simulink model "total"  (R2021a)
settings: Solver=VariableStepAuto  StartTime=0.0  StopTime=2.5  RelTol=1e-3
undefined symbols (not defined in the file or in its folder): Ion, Lithium
libraries: pid_lib x7, spsSeriesRLCBranchLib x4, spsMeanLib x4, spsACVoltageSourceLib x3, spsThreePhaseSeriesRLCBranchLib x3, spsGroundLib x2, spsabctodq0Lib x2, eePwmGenerator x2, spsOnDelayLib x2, spsBatteryLib x2, spsCurrentMeasurementLib x1, spsDiodeLib x1
settings Model: Creator=XieWHirlwind_TB  LastModifiedBy=XieWHirlwind_TB

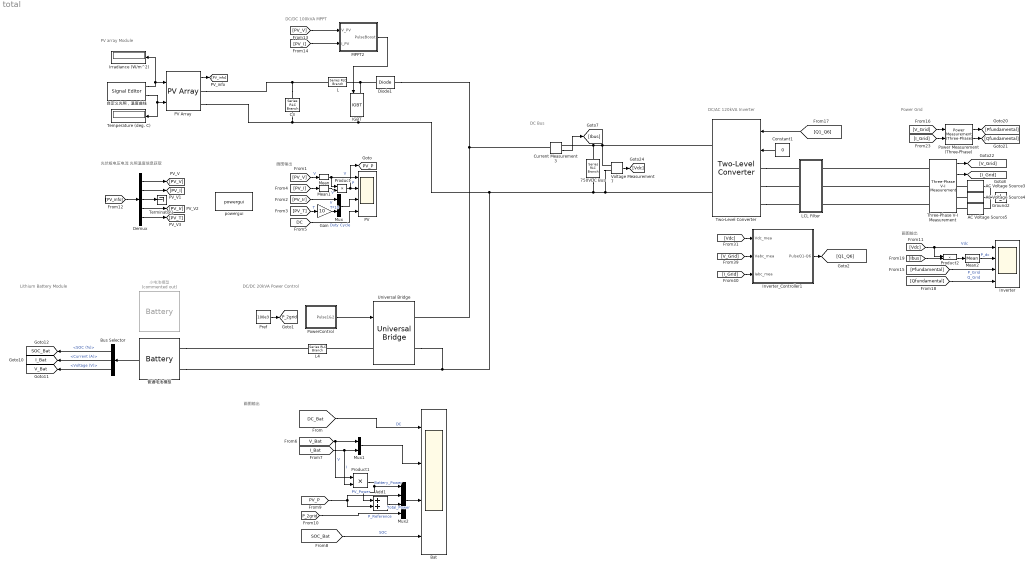
== system total ==
  note: 光伏板电压电流
      | 光照温度信息获取
  note: PV array Module
  note: 画图输出
  note: DC/DC 100kVA MPPT
  note: 画图输出
  note: DC/DC 20kVA Power Control
  note: Lithium Battery Module
  note: 画图输出
  note: DC/AC 120kVA Inverter
  note: Power Grid
  note: DC Bus
  750VDC Bus : spsSeriesRLCBranchLib/Series RLC Branch  LConnTagsString=__new0  RConnTagsString=__new0  BranchType=C  Resistance=1  Inductance=1e-3  SetiL0=off  InitialCurrent=0  Capacitance=470e-6  Setx0=on  InitialVoltage=0  Measurements=None
  AC Voltage Source3 : spsACVoltageSourceLib/AC Voltage Source  Amplitude=220*sqrt(2)  Phase=0  Frequency=50  SampleTime=0  Measurements=None  BusType=swing  Pref=10e3  Qref=0  Qmin=-inf  Qmax=+inf
  AC Voltage Source4 : spsACVoltageSourceLib/AC Voltage Source  Amplitude=220*sqrt(2)  Phase=-120  Frequency=50  SampleTime=0  Measurements=None  BusType=swing  Pref=10e3  Qref=0  Qmin=-inf  Qmax=+inf
  AC Voltage Source5 : spsACVoltageSourceLib/AC Voltage Source  Amplitude=220*sqrt(2)  Phase=120  Frequency=50  SampleTime=0  Measurements=None  BusType=swing  Pref=10e3  Qref=0  Qmin=-inf  Qmax=+inf
  Add1 : Sum
  Bat : Scope  NumInputPorts=4
  Bus Selector : BusSelector  OutputSignals=SOC (%),Current (A),Voltage (V)
  C3 : spsSeriesRLCBranchLib/Series RLC Branch  LConnTagsString=__new0  RConnTagsString=__new0  BranchType=C  Resistance=1.0  Inductance=1.0  SetiL0=off  InitialCurrent=0  Capacitance=470e-6  Setx0=off  InitialVoltage=0  Measurements=Branch voltage
  Constant1 : Constant  Value=0
  Current Measurement3 : spsCurrentMeasurementLib/Current Measurement  PhasorSimulation=off  OutputType=Complex  PSBequivalent=0
  Demux : Demux  Outputs=5
  Diode1 : spsDiodeLib/Diode  Ron=1e-3  Lon=0  Vf=0.7  IC=0  UseSnubber=off  Rs=inf  Cs=inf  Measurements=off
  Gain : Gain  Gain=10
  Ground2 : spsGroundLib/Ground  LConnTagsString=a
  IGBT : spsIGBTLib/IGBT  Ron=1e-3  Lon=0  Vf=0.7  Tf=1e-6  Tt=2e-6  IC=0  Rs=1e5  Cs=inf  Measurements=off
  Inverter : Scope  NumInputPorts=4
  Inverter_Controller1 : Subsystem  mask{Kp_Vdc_regulator=0.1, Ki_Vdc_regulator=10, Kp_Vdc_control=1, Ki_Vdc_control=1000, Kp_Q_regulator=1e-3, Ki_Q_regulator=1, Ts_Control=1e-4, L12=1e-3+3e-6, fsw=10e3, Vdc=750, Q_ref=5e3}
      mask prompts: Kp_Vdc_regulator "Kp"; Ki_Vdc_regulator "Ki"; Kp_Vdc_control "Kp"; Ki_Vdc_control "Ki"; Kp_Q_regulator "Kp"; Ki_Q_regulator "Ki"; Ts_Control "PI控制器控制周期(s)"; L12 "滤波器总串联电感(H)"; fsw "PWM频率(Hz)"; Vdc "直流母线电压(V)"; Q_ref "无功功率(VA)"
      mask DialogControl Container3 Prompt: 直流母线电压控制
      mask DialogControl Container4 Prompt: 电流环控制
      mask DialogControl Container5 Prompt: 无功功率控制
  Irradiance (W/m^2) : Display
      settings: Format=bank  Decimation=1000
  L : spsSeriesRLCBranchLib/Series RLC Branch  LConnTagsString=__new0  RConnTagsString=__new0  BranchType=RL  Resistance=0.0005  Inductance=1e-3  SetiL0=off  InitialCurrent=0  Capacitance=1e-6  Setx0=off  InitialVoltage=0  Measurements=None
  L4 : spsSeriesRLCBranchLib/Series RLC Branch  LConnTagsString=__new0  RConnTagsString=__new0  BranchType=RL  Resistance=0.001  Inductance=1e-3  SetiL0=off  InitialCurrent=0  Capacitance=1e-6  Setx0=off  InitialVoltage=0  Measurements=None
  LCL Filter : Subsystem  mask(LCL_Filter){Linv_LCL=1e-3, Lgrid_LCL=3e-6, Cap_LCL=1e-3, Rsnubber_LCL=0}
      mask prompts: Linv_LCL "逆变器侧电感"; Lgrid_LCL "电网侧电感"; Cap_LCL "并联电容"; Rsnubber_LCL "与电容串联的阻尼电阻"
  MPPT2 : Subsystem
  Mean : spsMeanLib/Mean  Freq=1e3  Vinit=0  Ts=1e-4
  Mean1 : spsMeanLib/Mean  Freq=1e3  Vinit=0  Ts=1e-4
  Mean2 : spsMeanLib/Mean  Freq=1/1e-3  Vinit=0  Ts=2e-6
  Mux : Mux  Inputs=2
  Mux1 : Mux  Inputs=2
  Mux2 : Mux
  PV : Scope  NumInputPorts=4
  PV Array : spsPVArrayLib/PV Array  Npar=45  Nser=10  PlotType=array @ 25 deg.C & specified irradiances  S_vec="[ 1000 800 350  100 ]"  Temp_C_vec="[ 45 25  ]"  ModuleName=A2Peak Power POWER ON P220-6x10  PlotWhenSelected=off  Pm=219.978  Ncell=60  Voc=36.72  Isc=7.98  Vm=30.3  Im=7.26  beta_Voc_pc=-0.35  alpha_Isc_pc=0.05  beta_Voc=-0.12852  alpha_Isc=0.00399  IL=8.0041  I0=1.8441e-10  nI=0.97472  Rsh=85.0716  Rs=0.25728  RobustModel=off  RobustCellTemperature=313.3991  BAL=on  Tc=1e-6  Tfilter=5e-5
  Power Measurement (Three-Phase) : eePowerMeasurement/Power Measurement (Three-Phase)  LabelModeActiveChoice=Discrete  F=50  K=[1]  Seq=Positive  Ts=1e-4
      settings: SourceProductBaseCode=PS
  PowerControl : Subsystem
  Pref : Constant  Value=100e3
  Product : Product
  Product1 : Product
  Product2 : Product
  Temperature (deg. C) : Display
      settings: Format=bank  Decimation=1000
  Terminator1 : Terminator
  Three-Phase V-I Measurement : spsThreePhaseVIMeasurementLib/Three-Phase V-I Measurement  VoltageMeasurement=phase-to-ground  SetLabelV=off  LabelV=Vabc  Vpu=off  VpuLL=off  CurrentMeasurement=yes  SetLabelI=off  LabelI=Iabc  Ipu=off  Pbase=100e6  Vbase=500e3  OutputType=Complex  PhasorSimulation=off  PSBequivalent=0
  Two-Level Converter : spsTwoLevelConverterLib/Two-Level Converter  ModelType=Switching devices  Ron=1e-3  Rs=1e6  Cs=inf  Vforward=[0,0]  Ron_Diode=1e-3  Rs_Diode=1e6  Cs_Diode=inf  Vf_Diode=1e-3  Rs_CurrentSource=inf
      settings: SourceProductBaseCode=PS
  Universal Bridge : spsUniversalBridgeLib/Universal Bridge  Arms=1  SnubberResistance=1e5  SnubberCapacitance=inf  Device=IGBT / Diodes  Ron=1e-3  Lon=0  ForwardVoltages="[0.7  0.7]"  ForwardVoltage=0  GTOparameters=[ 10e-6 , 20e-6 ]  IGBTparameters=[ 1e-6 , 2e-6 ]  Measurements=None  Measurements_2=None  converterType=Rectifier
  Voltage Measurement7 : spsVoltageMeasurementLib/Voltage Measurement  PhasorSimulation=off  OutputType=Complex  PSBequivalent=0
  powergui : spspowerguiLib/powergui  Priority=1  SimulationMode=Discrete  SampleTime=2e-6  frequency=60  Iterations=50  frequencyindice=0  Pbase=100e6  ErrMax=1e-4  UnitsV=kV  UnitsW=MW  buscounter=0  FunctionMessages=off  echomessages=off  EnableUseOfTLC=off  CurrentSourceSwitches=off  DisableSnubberDevices=off  DisableRonSwitches=off  DisableVfSwitches=off  DisplayEquations=off  AutomaticDiscreteSolvers=off  SolverType=Tustin/Backward Euler (TBE)  Interpol=off  ExternalGateDelay=off  methode=off  Ts=100  x0status=blocks  SPID=on  SwTol=0  HookPort=off  NonlinearTolerance=1e-4  nMaxIteration=100  ContinueOnMaxIteration=off  RestoreLinks=warning  ResistiveCurrentMeasurement=off  Frange=[0:2:500]  Ylog=off  Xlog=on  ShowGrid=off  save=off  variable=ZData  structure=0  ZoomFFT=off  StartTime=0.0  cycles=1  DisplayStyle=1  fundamental=60  FreqAxis=off  MaxFrequency=1000  frequencyindicesteady=1  RmsSteady=1  display=off
  小电池模型 : spsBatteryLib/Battery  Commented=on  BatType=Lithium-Ion  ShowTempParam=off  ThermalPreset=no  ShowAgeParam=off  NomV=640  NomQ=62.5/1000  SOC=50  Batt_Tr=30  PresetModel=off  MaxQ=62.5/100000  MinV=480  FullV=744.9518  Dis_rate=27.1739  R=0.1024  Normal_OP=56.5217/100000  expZone="[691.4469      3.070652/100000]"  current=[6.5 13 32.5]  Units=Time  Tci=20  NomT=20  T2=-30  MaxQ2=4.8  FullV2=7.1  Normal_OP2=5.655  expZone2="[6.58           1]"  Rca=0.6  ti=2000  Dp=0  Neq0=0  Tsim=1e6  Ta1=25  Qeol=5.4*0.9  Reol=0.013333*1.2  Char_age=[2.3478, 3]  Dis_age=[2.3478, 10]  N1=1500  N2=10500  N3=1000  N4=1400  Ta2=45  N5=950
  普通电池模型 : spsBatteryLib/Battery  BatType=Lithium-Ion  ShowTempParam=off  ThermalPreset=no  ShowAgeParam=off  NomV=640  NomQ=62.5  SOC=50  Batt_Tr=30  PresetModel=on  MaxQ=62.5  MinV=480  FullV=744.9518  Dis_rate=27.1739  R=0.1024  Normal_OP=56.5217  expZone="[691.4469      3.070652]"  current=[6.5 13 32.5]  Units=Time  Tci=20  NomT=20  T2=-30  MaxQ2=4.8  FullV2=7.1  Normal_OP2=5.655  expZone2="[6.58           1]"  Rca=0.6  ti=2000  Dp=0  Neq0=0  Tsim=1e6  Ta1=25  Qeol=5.4*0.9  Reol=0.013333*1.2  Char_age=[2.3478, 3]  Dis_age=[2.3478, 10]  N1=1500  N2=10500  N3=1000  N4=1400  Ta2=45  N5=950
  自定义光照，温度曲线 : SignalEditorBlockLib/Signal Editor  FileName=Irr_Temp_1.mat  ActiveScenario=Scenario  ActiveSignal=Temp  IsBus=off  OutputBusObjectStr=Bus: BusObject  SampleTime=0  ZeroCross=off  OutputAfterFinalValue=Setting to zero  Unit=inherit  PreserveSignalName=on
  tag scope: I_Bat=global, PV_P=global, P_2grid=global, SOC_Bat=global, V_Bat=global
  wires:
  Demux/4 -> [PV_Ir]
  [DC] -> PV/4  "Duty Cycle"
  [PV_V] -> MPPT2/1(V_PV)
  [PV_V] -> Mean/1  "V"
  Gain/1 -> Mux/2  "T*10"
  [PV_T] -> Gain/1  "T"
  Demux/5 -> [PV_T]
  Mean/1 -> Product/1, PV/1  "V"
  [PV_I] -> Mean1/1
  [PV_info] -> Demux/1
  MPPT2/1(PulseBoost) -> IGBT/1
  Demux/2 -> [PV_I]
  自定义光照，温度曲线/2 -> Temperature (deg. C)/1, PV Array/2
  Demux/3 -> Terminator1/1
  Mean1/1 -> Product/2  "V"
  Product/1 -> [PV_P], PV/2  "P"
  Demux/1 -> [PV_V]
  [PV_Ir] -> Mux/1  "Ir"
  自定义光照，温度曲线/1 -> Irradiance (W/m^2)/1, PV Array/1
  Mux/1 -> PV/3
  [PV_I] -> MPPT2/2(I_PV)
  PV Array/1 -> [PV_info]
  Pref/1 -> [P_2grid]
  PowerControl/1(Pulse1&2) -> Universal Bridge/1
  Mux1/1 -> Bat/2
  [PV_P] -> Add1/2, Mux2/2  "PV_Power"
  [I_Bat] -> Product1/2, Mux1/2  "I"
  [V_Bat] -> Mux1/1, Product1/1  "V"
  [DC_Bat] -> Bat/1  "DC"
  Bus Selector/3 -> [V_Bat]  "<Voltage (V)>"
  Bus Selector/1 -> [SOC_Bat]  "<SOC (%)>"
  普通电池模型/1 -> Bus Selector/1
  Product1/1 -> Add1/1, Mux2/1  "Battery_Power"
  Bus Selector/2 -> [I_Bat]  "<Current (A)>"
  [SOC_Bat] -> Bat/4  "SOC"
  [P_2grid] -> Mux2/4  "P_Reference"
  Mux2/1 -> Bat/3
  Add1/1 -> Mux2/3  "Total_Power"
  Mean2/1 -> Inverter/2  "P_dc"
  Product2/1 -> Mean2/1
  Three-Phase V-I Measurement/1 -> [V_Grid]
  [Vdc] -> Inverter_Controller1/1(Vdc_mea)
  Power Measurement (Three-Phase)/1 -> [Pfundamental]
  [Vdc] -> Inverter/1, Product2/1  "Vdc"
  [I_Grid] -> Power Measurement (Three-Phase)/2
  Three-Phase V-I Measurement/2 -> [I_Grid]
  [Qfundamental] -> Inverter/4  "Q_Grid"
  Power Measurement (Three-Phase)/2 -> [Qfundamental]
  [I_Grid] -> Inverter_Controller1/3(Iabc_mea)
  [Pfundamental] -> Inverter/3  "P_Grid"
  [Q1_Q6] -> Two-Level Converter/1
  [V_Grid] -> Power Measurement (Three-Phase)/1
  Constant1/1 -> Two-Level Converter/2
  [V_Grid] -> Inverter_Controller1/2(Vabc_mea)
  Inverter_Controller1/1(PulseQ1-Q6) -> [Q1_Q6]
  [Ibus] -> Product2/2
  Voltage Measurement7/1 -> [Vdc]
  Current Measurement3/1 -> [Ibus]
  connections:
  Diode1/LConn1 -- L/RConn1 -- IGBT/LConn1
  C3/LConn1 -- PV Array/RConn1 -- L/LConn1
  Universal Bridge/LConn1 -- L4/RConn1
  普通电池模型/LConn1 -- L4/LConn1
  Ground2/LConn1 -- AC Voltage Source5/LConn1 -- AC Voltage Source4/LConn1 -- AC Voltage Source3/LConn1
  Two-Level Converter/LConn3 -- LCL Filter/LConn3
  AC Voltage Source5/RConn1 -- Three-Phase V-I Measurement/RConn3
  Two-Level Converter/LConn2 -- LCL Filter/LConn2
  AC Voltage Source3/RConn1 -- Three-Phase V-I Measurement/RConn1
  Three-Phase V-I Measurement/LConn1 -- LCL Filter/RConn1
  Three-Phase V-I Measurement/LConn2 -- LCL Filter/RConn2
  Three-Phase V-I Measurement/LConn3 -- LCL Filter/RConn3
  AC Voltage Source4/RConn1 -- Three-Phase V-I Measurement/RConn2
  Two-Level Converter/LConn1 -- LCL Filter/LConn1
  PV Array/RConn2 -- Two-Level Converter/RConn2 -- Voltage Measurement7/LConn2 -- 750VDC Bus/RConn1 -- 普通电池模型/LConn2 -- Universal Bridge/RConn2 -- IGBT/RConn1 -- C3/RConn1
  Voltage Measurement7/LConn1 -- 750VDC Bus/LConn1 -- Current Measurement3/RConn1 -- Two-Level Converter/RConn1
  Current Measurement3/LConn1 -- Diode1/RConn1 -- Universal Bridge/RConn1

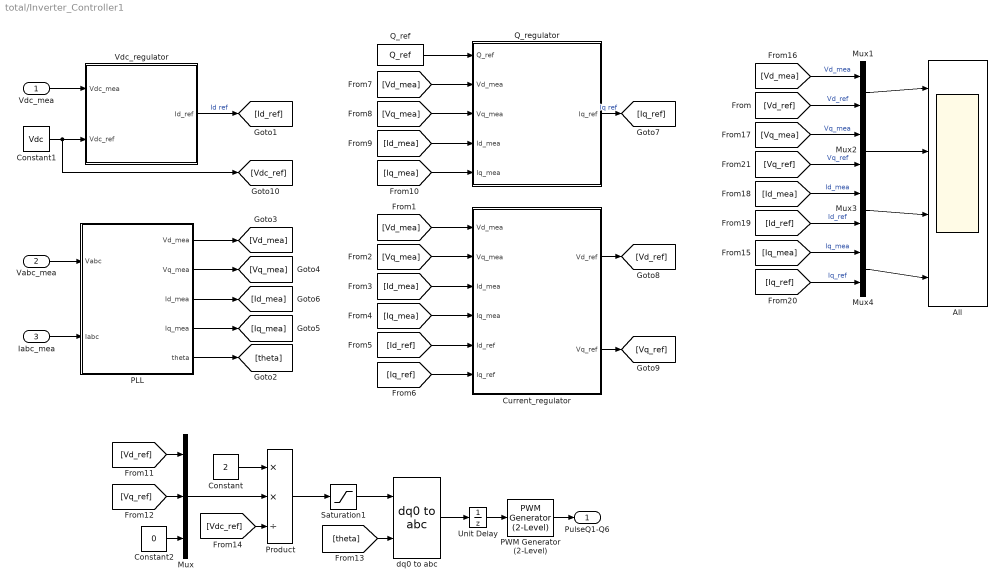
== system total/Inverter_Controller1 ==
  Vdc_mea : Inport
  Vabc_mea : Inport  Port=2
  Iabc_mea : Inport  Port=3
  All : Scope  NumInputPorts=4
  Constant : Constant  Value=2
  Constant1 : Constant  Value=Vdc
  Constant2 : Constant  Value=0
  Current_regulator : Subsystem
  Mux : Mux  Inputs=3
  Mux{1..4} (4 alike) : Mux  Inputs=2
  PLL : Subsystem
  PWM Generator (2-Level) : spsPWMGenerator2LevelLib/PWM Generator (2-Level)  ModulatorType=Three-phase bridge (6 pulses)  ModulatorMode=Unsynchronized  Fc=fsw  Pc=90  nF=27  MinMax="[ -1  1 ]"  SamplingTechnique=Asymmetrical regular (double edge)  ModulatingSignals=off  m=0.8  Freq=60  Phase=0  Ts=1e-6  ShowCarrierOutport=off
  Product : Product  Inputs=**/
  Q_ref : Constant  Value=Q_ref
  Q_regulator : Subsystem
  Saturation1 : Saturate  UpperLimit=2  LowerLimit=-2
  Unit Delay : UnitDelay  SampleTime=Ts_Control  HasFrameUpgradeWarning=on
  Vdc_regulator : Subsystem
  dq0 to abc : spsdq0toabcLib/dq0 to abc  Alignment=90 degrees behind phase A axis
  PulseQ1-Q6 : Outport
  wires:
  Constant1/1 -> [Vdc_ref], Vdc_regulator/2(Vdc_ref)
  Vabc_mea/1 -> PLL/1(Vabc)
  Iabc_mea/1 -> PLL/2(Iabc)
  PWM Generator (2-Level)/1 -> PulseQ1-Q6/1
  Saturation1/1 -> dq0 to abc/1
  dq0 to abc/1 -> Unit Delay/1
  Product/1 -> Saturation1/1
  Unit Delay/1 -> PWM Generator (2-Level)/1
  Vdc_mea/1 -> Vdc_regulator/1(Vdc_mea)
  Q_ref/1 -> Q_regulator/1(Q_ref)
  Constant/1 -> Product/1
  [Vdc_ref] -> Product/3
  Vdc_regulator/1(Id_ref) -> [Id_ref]  "Id ref"
  PLL/5(theta) -> [theta]
  PLL/1(Vd_mea) -> [Vd_mea]
  PLL/2(Vq_mea) -> [Vq_mea]
  PLL/3(Id_mea) -> [Id_mea]
  PLL/4(Iq_mea) -> [Iq_mea]
  [Vd_mea] -> Current_regulator/1(Vd_mea)
  [Vq_mea] -> Current_regulator/2(Vq_mea)
  [Id_mea] -> Current_regulator/3(Id_mea)
  [Iq_mea] -> Current_regulator/4(Iq_mea)
  [Id_ref] -> Current_regulator/5(Id_ref)
  Q_regulator/1(Iq_ref) -> [Iq_ref]  "Iq ref"
  [Iq_ref] -> Current_regulator/6(Iq_ref)
  [Vd_mea] -> Q_regulator/2(Vd_mea)
  [Vq_mea] -> Q_regulator/3(Vq_mea)
  [Id_mea] -> Q_regulator/4(Id_mea)
  [Iq_mea] -> Q_regulator/5(Iq_mea)
  Current_regulator/1(Vd_ref) -> [Vd_ref]
  Current_regulator/2(Vq_ref) -> [Vq_ref]
  [Vd_ref] -> Mux/1
  [Vq_ref] -> Mux/2
  Constant2/1 -> Mux/3
  Mux/1 -> Product/2
  [theta] -> dq0 to abc/2
  [Vd_mea] -> Mux1/1  "Vd_mea"
  [Vd_ref] -> Mux1/2  "Vd_ref"
  [Vq_mea] -> Mux2/1  "Vq_mea"
  [Vq_ref] -> Mux2/2  "Vq_ref"
  [Id_mea] -> Mux3/1  "Id_mea"
  [Id_ref] -> Mux3/2  "Id_ref"
  [Iq_mea] -> Mux4/1  "Iq_mea"
  [Iq_ref] -> Mux4/2  "Iq_ref"
  Mux2/1 -> All/2
  Mux1/1 -> All/1
  Mux3/1 -> All/3
  Mux4/1 -> All/4

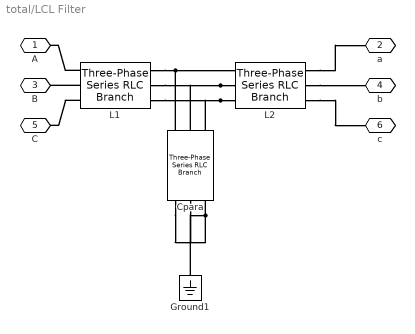
== system total/LCL Filter ==
  Cpara : spsThreePhaseSeriesRLCBranchLib/Three-Phase Series RLC Branch  LConnTagsString=A|B|C  RConnTagsString=A|B|C  BranchType=RC  Resistance=Rsnubber_LCL  Inductance=1e-3  Capacitance=Cap_LCL  Measurements=None
  Ground1 : spsGroundLib/Ground  LConnTagsString=a
  L1 : spsThreePhaseSeriesRLCBranchLib/Three-Phase Series RLC Branch  LConnTagsString=A|B|C  RConnTagsString=A|B|C  BranchType=L  Resistance=1  Inductance=Linv_LCL  Capacitance=1e-6  Measurements=None
  L2 : spsThreePhaseSeriesRLCBranchLib/Three-Phase Series RLC Branch  LConnTagsString=A|B|C  RConnTagsString=A|B|C  BranchType=L  Resistance=1  Inductance=Lgrid_LCL  Capacitance=1e-6  Measurements=None
  A : PMIOPort  Side=Left
  a : PMIOPort  Port=2  Side=Right
  B : PMIOPort  Port=3  Side=Left
  b : PMIOPort  Port=4  Side=Right
  C : PMIOPort  Port=5  Side=Left
  c : PMIOPort  Port=6  Side=Right
  connections:
  L2/RConn2 -- b/RConn1
  L2/LConn2 -- L1/RConn2 -- Cpara/LConn2
  L2/LConn3 -- L1/RConn3 -- Cpara/LConn3
  Cpara/RConn3 -- Cpara/RConn2 -- Ground1/LConn1 -- Cpara/RConn1
  L1/LConn3 -- C/RConn1
  L1/LConn1 -- A/RConn1
  L2/RConn1 -- a/RConn1
  L1/LConn2 -- B/RConn1
  L2/RConn3 -- c/RConn1
  L1/RConn1 -- L2/LConn1 -- Cpara/LConn1

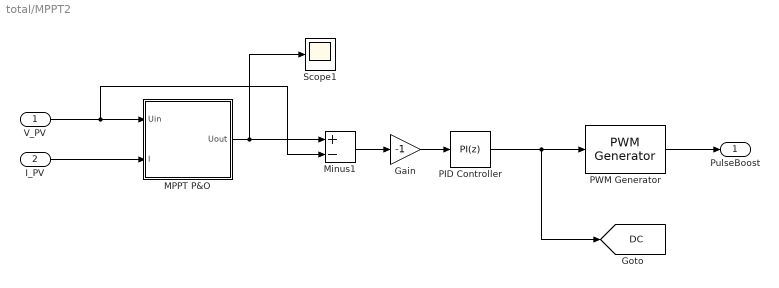
== system total/MPPT2 ==
  V_PV : Inport
  I_PV : Inport  Port=2
  Gain : Gain  Gain=-1
  MPPT P&O : Subsystem
  Minus1 : Sum  Inputs=+-
  PID Controller : pid_lib/PID Controller  Controller=PI  Form=Parallel  TimeDomain=Discrete-time  UseExternalTs=off  SampleTime=1e-4  IntegratorMethod=Forward Euler  FilterMethod=Forward Euler  ControllerParametersSource=internal  P=0.001  I=0.1  D=0  UseFilter=on  N=100  TunerSelectOption=Transfer Function Based (PID Tuner App)  InitialConditionSource=internal  InitialConditionForIntegrator=0  InitialConditionForFilter=0  DifferentiatorICPrevScaledInput=0  ExternalReset=none  TrackingMode=off  Kt=1  LimitOutput=on  SatLimitsSource=internal  UpperSaturationLimit=1  LowerSaturationLimit=0  LinearizeAsGain=on  AntiWindupMode=none  Kb=1  POutMin=[]  POutMax=[]  IOutMin=[]  IOutMax=[]  DOutMin=[]  DOutMax=[]  NOutMin=[]  NOutMax=[]  SumOutMin=[]  SumOutMax=[]  SaturationOutMin=[]  SaturationOutMax=[]  PParamMin=[]  PParamMax=[]  IParamMin=[]  IParamMax=[]  DParamMin=[]  DParamMax=[]  NParamMin=[]  NParamMax=[]  KbParamMin=[]  KbParamMax=[]  KtParamMin=[]  KtParamMax=[]  KbOutMin=[]  KbOutMax=[]  KtOutMin=[]  KtOutMax=[]  IntegratorOutMin=[]  IntegratorOutMax=[]  FilterOutMin=[]  FilterOutMax=[]  SumI1OutMin=[]  SumI1OutMax=[]  SumI2OutMin=[]  SumI2OutMax=[]  SumI3OutMin=[]  SumI3OutMax=[]  SumI4OutMin=[]  SumI4OutMax=[]  SumDOutMin=[]  SumDOutMax=[]  DifferentiatorOutMin=[]  DifferentiatorOutMax=[]  FilterDiffOutCoefMin=[]  FilterDiffOutCoefMax=[]  ReciprocalOutMin=[]  ReciprocalOutMax=[]  SumDenOutMin=[]  SumDenOutMax=[]  SumNumOutMin=[]  SumNumOutMax=[]  DivideOutMin=[]  DivideOutMax=[]  UdiffTsProdOutMin=[]  UdiffTsProdOutMax=[]  NTsProdOutMin=[]  NTsProdOutMax=[]  UintegralTsProdOutMin=[]  UintegralTsProdOutMax=[]  UngainTsProdOutMin=[]  UngainTsProdOutMax=[]  IntegratorContinuousStateAttributes=''  IntegratorStateMustResolveToSignalObject=off  IntegratorRTWStateStorageClass=Auto  FilterContinuousStateAttributes=''  FilterStateMustResolveToSignalObject=off  FilterRTWStateStorageClass=Auto  ParallelPVariant=InternalParameters  IdealPVariant=Disabled  IVariant=InternalParameters  DVariant=Disabled  IntegratorVariant=Discrete  SatVariant=Enabled  AWVariant=Passthrough  PCopyVariant=Disabled  TRVariant=Disabled  FdbkBlocksVariant=Forward  IdealPFdbkVariant=Disabled  SatFdbkVariant=Disabled  DerivativeFilterVariant=Disabled  NVariant=Disabled  NCopyVariant=Disabled_SignalSpec  FilterICVariant=Disabled  IntegratorICVariant=InternalICs  ExternalResetVariant=Disabled  TRSumVariant=Passthrough  SumFdbkVariant=Disabled  SumVariant=Sum_PI  TsampFilterVariant=InternalTs  TsampNgainVariant=Passthrough  TsampIntegralVariant=Passthrough  ExternalSaturationOutDataTypeStr=Inherit: Same as second input
  PWM Generator : eePwmGenerator/PWM Generator  CarrCount=Up  Tper=1e-4  Ts=2e-6
  Scope1 : Scope
  PulseBoost : Outport
  tag scope: DC=global
  wires:
  PWM Generator/1 -> PulseBoost/1
  I_PV/1 -> MPPT P&O/2(I)
  V_PV/1 -> Minus1/2, MPPT P&O/1(Uin)
  MPPT P&O/1(Uout) -> Minus1/1, Scope1/1
  Minus1/1 -> Gain/1
  PID Controller/1 -> [DC], PWM Generator/1
  Gain/1 -> PID Controller/1

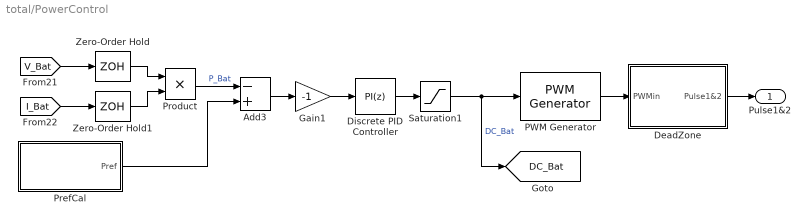
== system total/PowerControl ==
  Add3 : Sum  Inputs=-+
  DeadZone : Subsystem
  Discrete PID Controller : pid_lib/PID Controller  Controller=PI  Form=Parallel  TimeDomain=Discrete-time  UseExternalTs=off  SampleTime=1e-4  IntegratorMethod=Forward Euler  FilterMethod=Forward Euler  ControllerParametersSource=internal  P=2e-6  I=2e-3  D=0  UseFilter=on  N=100  TunerSelectOption=Transfer Function Based (PID Tuner App)  InitialConditionSource=internal  InitialConditionForIntegrator=0.8  InitialConditionForFilter=0  DifferentiatorICPrevScaledInput=0  ExternalReset=none  TrackingMode=off  Kt=1  LimitOutput=off  SatLimitsSource=internal  UpperSaturationLimit=1  LowerSaturationLimit=0  LinearizeAsGain=off  AntiWindupMode=none  Kb=1  POutMin=[]  POutMax=[]  IOutMin=[]  IOutMax=[]  DOutMin=[]  DOutMax=[]  NOutMin=[]  NOutMax=[]  SumOutMin=[]  SumOutMax=[]  SaturationOutMin=[]  SaturationOutMax=[]  PParamMin=[]  PParamMax=[]  IParamMin=[]  IParamMax=[]  DParamMin=[]  DParamMax=[]  NParamMin=[]  NParamMax=[]  KbParamMin=[]  KbParamMax=[]  KtParamMin=[]  KtParamMax=[]  KbOutMin=[]  KbOutMax=[]  KtOutMin=[]  KtOutMax=[]  IntegratorOutMin=[]  IntegratorOutMax=[]  FilterOutMin=[]  FilterOutMax=[]  SumI1OutMin=[]  SumI1OutMax=[]  SumI2OutMin=[]  SumI2OutMax=[]  SumI3OutMin=[]  SumI3OutMax=[]  SumI4OutMin=[]  SumI4OutMax=[]  SumDOutMin=[]  SumDOutMax=[]  DifferentiatorOutMin=[]  DifferentiatorOutMax=[]  FilterDiffOutCoefMin=[]  FilterDiffOutCoefMax=[]  ReciprocalOutMin=[]  ReciprocalOutMax=[]  SumDenOutMin=[]  SumDenOutMax=[]  SumNumOutMin=[]  SumNumOutMax=[]  DivideOutMin=[]  DivideOutMax=[]  UdiffTsProdOutMin=[]  UdiffTsProdOutMax=[]  NTsProdOutMin=[]  NTsProdOutMax=[]  UintegralTsProdOutMin=[]  UintegralTsProdOutMax=[]  UngainTsProdOutMin=[]  UngainTsProdOutMax=[]  IntegratorContinuousStateAttributes=''  IntegratorStateMustResolveToSignalObject=off  IntegratorRTWStateStorageClass=Auto  FilterContinuousStateAttributes=''  FilterStateMustResolveToSignalObject=off  FilterRTWStateStorageClass=Auto  ParallelPVariant=InternalParameters  IdealPVariant=Disabled  IVariant=InternalParameters  DVariant=Disabled  IntegratorVariant=Discrete  SatVariant=Disabled  AWVariant=Passthrough  PCopyVariant=Disabled  TRVariant=Disabled  FdbkBlocksVariant=Forward  IdealPFdbkVariant=Disabled  SatFdbkVariant=Disabled  DerivativeFilterVariant=Disabled  NVariant=Disabled  NCopyVariant=Disabled_SignalSpec  FilterICVariant=Disabled  IntegratorICVariant=InternalICs  ExternalResetVariant=Disabled  TRSumVariant=Passthrough  SumFdbkVariant=Disabled  SumVariant=Sum_PI  TsampFilterVariant=InternalTs  TsampNgainVariant=Passthrough  TsampIntegralVariant=Passthrough  ExternalSaturationOutDataTypeStr=Inherit: Same as second input
  Gain1 : Gain  Gain=-1
  PWM Generator : eePwmGenerator/PWM Generator  CarrCount=Up  Tper=1e-4  Ts=2e-6
  PrefCal : Subsystem
  Product : Product
  Saturation1 : Saturate  UpperLimit=0.98  LowerLimit=0
  Zero-Order Hold : ZeroOrderHold  SampleTime=1e-4
  Zero-Order Hold1 : ZeroOrderHold  SampleTime=1e-4
  Pulse1&2 : Outport
  tag scope: DC_Bat=global
  wires:
  Zero-Order Hold1/1 -> Product/2
  Zero-Order Hold/1 -> Product/1
  Gain1/1 -> Discrete PID Controller/1
  Add3/1 -> Gain1/1
  Saturation1/1 -> PWM Generator/1, [DC_Bat]  "DC_Bat"
  Discrete PID Controller/1 -> Saturation1/1
  Product/1 -> Add3/1  "P_Bat"
  [I_Bat] -> Zero-Order Hold1/1
  [V_Bat] -> Zero-Order Hold/1
  PWM Generator/1 -> DeadZone/1(PWMin)
  DeadZone/1(Pulse1&2) -> Pulse1&2/1
  PrefCal/1(Pref) -> Add3/2

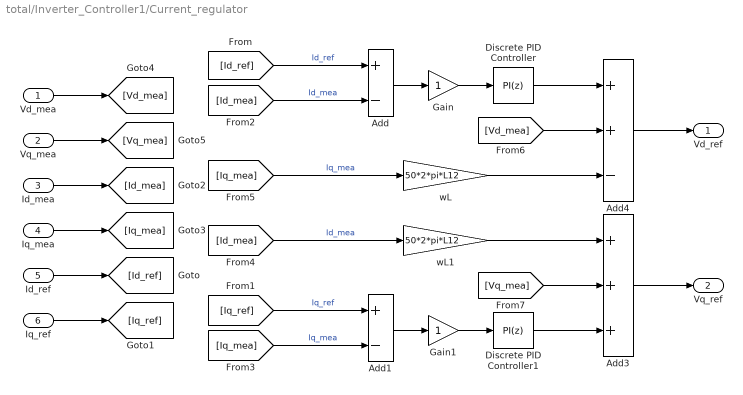
== system total/Inverter_Controller1/Current_regulator ==
  Vd_mea : Inport
  Vq_mea : Inport  Port=2
  Id_mea : Inport  Port=3
  Iq_mea : Inport  Port=4
  Id_ref : Inport  Port=5
  Iq_ref : Inport  Port=6
  Add : Sum  Inputs=+-
  Add1 : Sum  Inputs=+-
  Add3 : Sum  Inputs=+++
  Add4 : Sum  Inputs=++-
  Discrete PID Controller : pid_lib/PID Controller  Controller=PI  Form=Parallel  TimeDomain=Discrete-time  UseExternalTs=off  SampleTime=Ts_Control  IntegratorMethod=Forward Euler  FilterMethod=Forward Euler  ControllerParametersSource=internal  P=1.7  I=Ki_Vdc_control  D=0  UseFilter=on  N=100  TunerSelectOption=Transfer Function Based (PID Tuner App)  InitialConditionSource=internal  InitialConditionForIntegrator=0  InitialConditionForFilter=0  DifferentiatorICPrevScaledInput=0  ExternalReset=none  TrackingMode=off  Kt=1  LimitOutput=off  SatLimitsSource=internal  UpperSaturationLimit=inf  LowerSaturationLimit=-inf  LinearizeAsGain=off  AntiWindupMode=none  Kb=1  POutMin=[]  POutMax=[]  IOutMin=[]  IOutMax=[]  DOutMin=[]  DOutMax=[]  NOutMin=[]  NOutMax=[]  SumOutMin=[]  SumOutMax=[]  SaturationOutMin=[]  SaturationOutMax=[]  PParamMin=[]  PParamMax=[]  IParamMin=[]  IParamMax=[]  DParamMin=[]  DParamMax=[]  NParamMin=[]  NParamMax=[]  KbParamMin=[]  KbParamMax=[]  KtParamMin=[]  KtParamMax=[]  KbOutMin=[]  KbOutMax=[]  KtOutMin=[]  KtOutMax=[]  IntegratorOutMin=[]  IntegratorOutMax=[]  FilterOutMin=[]  FilterOutMax=[]  SumI1OutMin=[]  SumI1OutMax=[]  SumI2OutMin=[]  SumI2OutMax=[]  SumI3OutMin=[]  SumI3OutMax=[]  SumI4OutMin=[]  SumI4OutMax=[]  SumDOutMin=[]  SumDOutMax=[]  DifferentiatorOutMin=[]  DifferentiatorOutMax=[]  FilterDiffOutCoefMin=[]  FilterDiffOutCoefMax=[]  ReciprocalOutMin=[]  ReciprocalOutMax=[]  SumDenOutMin=[]  SumDenOutMax=[]  SumNumOutMin=[]  SumNumOutMax=[]  DivideOutMin=[]  DivideOutMax=[]  UdiffTsProdOutMin=[]  UdiffTsProdOutMax=[]  NTsProdOutMin=[]  NTsProdOutMax=[]  UintegralTsProdOutMin=[]  UintegralTsProdOutMax=[]  UngainTsProdOutMin=[]  UngainTsProdOutMax=[]  IntegratorContinuousStateAttributes=''  IntegratorStateMustResolveToSignalObject=off  IntegratorRTWStateStorageClass=Auto  FilterContinuousStateAttributes=''  FilterStateMustResolveToSignalObject=off  FilterRTWStateStorageClass=Auto  ParallelPVariant=InternalParameters  IdealPVariant=Disabled  IVariant=InternalParameters  DVariant=Disabled  IntegratorVariant=Discrete  SatVariant=Disabled  AWVariant=Passthrough  PCopyVariant=Disabled  TRVariant=Disabled  FdbkBlocksVariant=Forward  IdealPFdbkVariant=Disabled  SatFdbkVariant=Disabled  DerivativeFilterVariant=Disabled  NVariant=Disabled  NCopyVariant=Disabled_SignalSpec  FilterICVariant=Disabled  IntegratorICVariant=InternalICs  ExternalResetVariant=Disabled  TRSumVariant=Passthrough  SumFdbkVariant=Disabled  SumVariant=Sum_PI  TsampFilterVariant=InternalTs  TsampNgainVariant=Passthrough  TsampIntegralVariant=Passthrough  ExternalSaturationOutDataTypeStr=Inherit: Same as second input
  Discrete PID Controller1 : pid_lib/PID Controller  Controller=PI  Form=Parallel  TimeDomain=Discrete-time  UseExternalTs=off  SampleTime=Ts_Control  IntegratorMethod=Forward Euler  FilterMethod=Forward Euler  ControllerParametersSource=internal  P=1.7  I=Ki_Vdc_control  D=0.1  UseFilter=on  N=100  TunerSelectOption=Transfer Function Based (PID Tuner App)  InitialConditionSource=internal  InitialConditionForIntegrator=0  InitialConditionForFilter=0  DifferentiatorICPrevScaledInput=0  ExternalReset=none  TrackingMode=off  Kt=1  LimitOutput=off  SatLimitsSource=internal  UpperSaturationLimit=inf  LowerSaturationLimit=-inf  LinearizeAsGain=off  AntiWindupMode=none  Kb=1  POutMin=[]  POutMax=[]  IOutMin=[]  IOutMax=[]  DOutMin=[]  DOutMax=[]  NOutMin=[]  NOutMax=[]  SumOutMin=[]  SumOutMax=[]  SaturationOutMin=[]  SaturationOutMax=[]  PParamMin=[]  PParamMax=[]  IParamMin=[]  IParamMax=[]  DParamMin=[]  DParamMax=[]  NParamMin=[]  NParamMax=[]  KbParamMin=[]  KbParamMax=[]  KtParamMin=[]  KtParamMax=[]  KbOutMin=[]  KbOutMax=[]  KtOutMin=[]  KtOutMax=[]  IntegratorOutMin=[]  IntegratorOutMax=[]  FilterOutMin=[]  FilterOutMax=[]  SumI1OutMin=[]  SumI1OutMax=[]  SumI2OutMin=[]  SumI2OutMax=[]  SumI3OutMin=[]  SumI3OutMax=[]  SumI4OutMin=[]  SumI4OutMax=[]  SumDOutMin=[]  SumDOutMax=[]  DifferentiatorOutMin=[]  DifferentiatorOutMax=[]  FilterDiffOutCoefMin=[]  FilterDiffOutCoefMax=[]  ReciprocalOutMin=[]  ReciprocalOutMax=[]  SumDenOutMin=[]  SumDenOutMax=[]  SumNumOutMin=[]  SumNumOutMax=[]  DivideOutMin=[]  DivideOutMax=[]  UdiffTsProdOutMin=[]  UdiffTsProdOutMax=[]  NTsProdOutMin=[]  NTsProdOutMax=[]  UintegralTsProdOutMin=[]  UintegralTsProdOutMax=[]  UngainTsProdOutMin=[]  UngainTsProdOutMax=[]  IntegratorContinuousStateAttributes=''  IntegratorStateMustResolveToSignalObject=off  IntegratorRTWStateStorageClass=Auto  FilterContinuousStateAttributes=''  FilterStateMustResolveToSignalObject=off  FilterRTWStateStorageClass=Auto  ParallelPVariant=InternalParameters  IdealPVariant=Disabled  IVariant=InternalParameters  DVariant=Disabled  IntegratorVariant=Discrete  SatVariant=Disabled  AWVariant=Passthrough  PCopyVariant=Disabled  TRVariant=Disabled  FdbkBlocksVariant=Forward  IdealPFdbkVariant=Disabled  SatFdbkVariant=Disabled  DerivativeFilterVariant=Disabled  NVariant=Disabled  NCopyVariant=Disabled_SignalSpec  FilterICVariant=Disabled  IntegratorICVariant=InternalICs  ExternalResetVariant=Disabled  TRSumVariant=Passthrough  SumFdbkVariant=Disabled  SumVariant=Sum_PI  TsampFilterVariant=InternalTs  TsampNgainVariant=Passthrough  TsampIntegralVariant=Passthrough  ExternalSaturationOutDataTypeStr=Inherit: Same as second input
  Gain : Gain
  Gain1 : Gain
  wL : Gain  Gain=50*2*pi*L12
  wL1 : Gain  Gain=50*2*pi*L12
  Vd_ref : Outport
  Vq_ref : Outport  Port=2
  wires:
  Vd_mea/1 -> [Vd_mea]
  [Id_ref] -> Add/1  "Id_ref"
  [Iq_ref] -> Add1/1  "Iq_ref"
  [Iq_mea] -> Add1/2  "Iq_mea"
  Add/1 -> Gain/1
  Gain/1 -> Discrete PID Controller/1
  Gain1/1 -> Discrete PID Controller1/1
  Add1/1 -> Gain1/1
  Id_mea/1 -> [Id_mea]
  Discrete PID Controller/1 -> Add4/1
  Discrete PID Controller1/1 -> Add3/3
  [Vq_mea] -> Add3/2
  Add4/1 -> Vd_ref/1
  Add3/1 -> Vq_ref/1
  [Id_mea] -> Add/2  "Id_mea"
  [Iq_mea] -> wL/1  "Iq_mea"
  [Id_mea] -> wL1/1  "Id_mea"
  wL1/1 -> Add3/1
  [Vd_mea] -> Add4/2
  wL/1 -> Add4/3
  Vq_mea/1 -> [Vq_mea]
  Iq_mea/1 -> [Iq_mea]
  Id_ref/1 -> [Id_ref]
  Iq_ref/1 -> [Iq_ref]

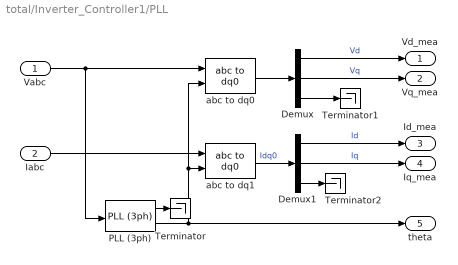
== system total/Inverter_Controller1/PLL ==
  Vabc : Inport
  Iabc : Inport  Port=2
  Demux : Demux  Outputs=3
  Demux1 : Demux  Outputs=3
  PLL (3ph) : spsPLL3phLib/PLL (3ph)  Fmin=45  Par_Init=[0 50]  ParK=[180, 3200, 1]  TcD=1e-4  MaxRateChangeFreq=12  FilterCutOffFreq=25  Ts=1e-4  AGC=on
  Terminator : Terminator
  Terminator1 : Terminator
  Terminator2 : Terminator
  abc to dq0 : spsabctodq0Lib/abc to dq0  Alignment=90 degrees behind phase A axis
  abc to dq1 : spsabctodq0Lib/abc to dq0  Alignment=90 degrees behind phase A axis
  Vd_mea : Outport
  Vq_mea : Outport  Port=2
  Id_mea : Outport  Port=3
  Iq_mea : Outport  Port=4
  theta : Outport  Port=5
  wires:
  Vabc/1 -> PLL (3ph)/1, abc to dq0/1
  PLL (3ph)/1 -> Terminator/1
  PLL (3ph)/2 -> abc to dq0/2, abc to dq1/2, theta/1
  abc to dq0/1 -> Demux/1
  Demux/1 -> Vd_mea/1  "Vd"
  Demux/2 -> Vq_mea/1  "Vq"
  Demux/3 -> Terminator1/1
  Iabc/1 -> abc to dq1/1
  Demux1/3 -> Terminator2/1
  Demux1/2 -> Iq_mea/1  "Iq"
  Demux1/1 -> Id_mea/1  "Id"
  abc to dq1/1 -> Demux1/1  "Idq0"

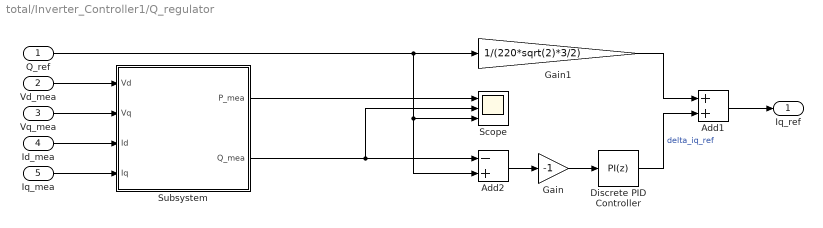
== system total/Inverter_Controller1/Q_regulator ==
  Q_ref : Inport
  Vd_mea : Inport  Port=2
  Vq_mea : Inport  Port=3
  Id_mea : Inport  Port=4
  Iq_mea : Inport  Port=5
  Add1 : Sum
  Add2 : Sum  Inputs=-+
  Discrete PID Controller : pid_lib/PID Controller  Controller=PI  Form=Parallel  TimeDomain=Discrete-time  UseExternalTs=off  SampleTime=-1  IntegratorMethod=Forward Euler  FilterMethod=Forward Euler  ControllerParametersSource=internal  P=Kp_Q_regulator  I=Ki_Q_regulator  D=0  UseFilter=on  N=100  TunerSelectOption=Transfer Function Based (PID Tuner App)  InitialConditionSource=internal  InitialConditionForIntegrator=0  InitialConditionForFilter=0  DifferentiatorICPrevScaledInput=0  ExternalReset=none  TrackingMode=off  Kt=1  LimitOutput=off  SatLimitsSource=internal  UpperSaturationLimit=inf  LowerSaturationLimit=-inf  LinearizeAsGain=off  AntiWindupMode=none  Kb=1  POutMin=[]  POutMax=[]  IOutMin=[]  IOutMax=[]  DOutMin=[]  DOutMax=[]  NOutMin=[]  NOutMax=[]  SumOutMin=[]  SumOutMax=[]  SaturationOutMin=[]  SaturationOutMax=[]  PParamMin=[]  PParamMax=[]  IParamMin=[]  IParamMax=[]  DParamMin=[]  DParamMax=[]  NParamMin=[]  NParamMax=[]  KbParamMin=[]  KbParamMax=[]  KtParamMin=[]  KtParamMax=[]  KbOutMin=[]  KbOutMax=[]  KtOutMin=[]  KtOutMax=[]  IntegratorOutMin=[]  IntegratorOutMax=[]  FilterOutMin=[]  FilterOutMax=[]  SumI1OutMin=[]  SumI1OutMax=[]  SumI2OutMin=[]  SumI2OutMax=[]  SumI3OutMin=[]  SumI3OutMax=[]  SumI4OutMin=[]  SumI4OutMax=[]  SumDOutMin=[]  SumDOutMax=[]  DifferentiatorOutMin=[]  DifferentiatorOutMax=[]  FilterDiffOutCoefMin=[]  FilterDiffOutCoefMax=[]  ReciprocalOutMin=[]  ReciprocalOutMax=[]  SumDenOutMin=[]  SumDenOutMax=[]  SumNumOutMin=[]  SumNumOutMax=[]  DivideOutMin=[]  DivideOutMax=[]  UdiffTsProdOutMin=[]  UdiffTsProdOutMax=[]  NTsProdOutMin=[]  NTsProdOutMax=[]  UintegralTsProdOutMin=[]  UintegralTsProdOutMax=[]  UngainTsProdOutMin=[]  UngainTsProdOutMax=[]  IntegratorContinuousStateAttributes=''  IntegratorStateMustResolveToSignalObject=off  IntegratorRTWStateStorageClass=Auto  FilterContinuousStateAttributes=''  FilterStateMustResolveToSignalObject=off  FilterRTWStateStorageClass=Auto  ParallelPVariant=InternalParameters  IdealPVariant=Disabled  IVariant=InternalParameters  DVariant=Disabled  IntegratorVariant=Discrete  SatVariant=Disabled  AWVariant=Passthrough  PCopyVariant=Disabled  TRVariant=Disabled  FdbkBlocksVariant=Forward  IdealPFdbkVariant=Disabled  SatFdbkVariant=Disabled  DerivativeFilterVariant=Disabled  NVariant=Disabled  NCopyVariant=Disabled_SignalSpec  FilterICVariant=Disabled  IntegratorICVariant=InternalICs  ExternalResetVariant=Disabled  TRSumVariant=Passthrough  SumFdbkVariant=Disabled  SumVariant=Sum_PI  TsampFilterVariant=InternalTs  TsampNgainVariant=Passthrough  TsampIntegralVariant=Passthrough  ExternalSaturationOutDataTypeStr=Inherit: Same as second input
  Gain : Gain  Gain=-1
  Gain1 : Gain  Gain=1/(220*sqrt(2)*3/2)
  Scope : Scope  NumInputPorts=3
  Subsystem : Subsystem
  Iq_ref : Outport
  wires:
  Q_ref/1 -> Add2/2, Scope/3, Gain1/1
  Gain1/1 -> Add1/1
  Discrete PID Controller/1 -> Add1/2  "delta_iq_ref"
  Add1/1 -> Iq_ref/1
  Subsystem/1(P_mea) -> Scope/1
  Subsystem/2(Q_mea) -> Add2/1, Scope/2
  Add2/1 -> Gain/1
  Gain/1 -> Discrete PID Controller/1
  Vd_mea/1 -> Subsystem/1(Vd)
  Vq_mea/1 -> Subsystem/2(Vq)
  Id_mea/1 -> Subsystem/3(Id)
  Iq_mea/1 -> Subsystem/4(Iq)

== system total/Inverter_Controller1/Vdc_regulator ==
  Vdc_mea : Inport
  Vdc_ref : Inport  Port=2
  Add : Sum  Inputs=+-
  Discrete PID Controller : pid_lib/PID Controller  Controller=PI  Form=Parallel  TimeDomain=Discrete-time  UseExternalTs=off  SampleTime=Ts_Control  IntegratorMethod=Forward Euler  FilterMethod=Forward Euler  ControllerParametersSource=internal  P=Kp_Vdc_regulator  I=Ki_Vdc_regulator  D=0  UseFilter=on  N=100  TunerSelectOption=Transfer Function Based (PID Tuner App)  InitialConditionSource=internal  InitialConditionForIntegrator=0  InitialConditionForFilter=0  DifferentiatorICPrevScaledInput=0  ExternalReset=none  TrackingMode=off  Kt=1  LimitOutput=off  SatLimitsSource=internal  UpperSaturationLimit=220  LowerSaturationLimit=-220  LinearizeAsGain=off  AntiWindupMode=none  Kb=1  POutMin=[]  POutMax=[]  IOutMin=[]  IOutMax=[]  DOutMin=[]  DOutMax=[]  NOutMin=[]  NOutMax=[]  SumOutMin=[]  SumOutMax=[]  SaturationOutMin=[]  SaturationOutMax=[]  PParamMin=[]  PParamMax=[]  IParamMin=[]  IParamMax=[]  DParamMin=[]  DParamMax=[]  NParamMin=[]  NParamMax=[]  KbParamMin=[]  KbParamMax=[]  KtParamMin=[]  KtParamMax=[]  KbOutMin=[]  KbOutMax=[]  KtOutMin=[]  KtOutMax=[]  IntegratorOutMin=[]  IntegratorOutMax=[]  FilterOutMin=[]  FilterOutMax=[]  SumI1OutMin=[]  SumI1OutMax=[]  SumI2OutMin=[]  SumI2OutMax=[]  SumI3OutMin=[]  SumI3OutMax=[]  SumI4OutMin=[]  SumI4OutMax=[]  SumDOutMin=[]  SumDOutMax=[]  DifferentiatorOutMin=[]  DifferentiatorOutMax=[]  FilterDiffOutCoefMin=[]  FilterDiffOutCoefMax=[]  ReciprocalOutMin=[]  ReciprocalOutMax=[]  SumDenOutMin=[]  SumDenOutMax=[]  SumNumOutMin=[]  SumNumOutMax=[]  DivideOutMin=[]  DivideOutMax=[]  UdiffTsProdOutMin=[]  UdiffTsProdOutMax=[]  NTsProdOutMin=[]  NTsProdOutMax=[]  UintegralTsProdOutMin=[]  UintegralTsProdOutMax=[]  UngainTsProdOutMin=[]  UngainTsProdOutMax=[]  IntegratorContinuousStateAttributes=''  IntegratorStateMustResolveToSignalObject=off  IntegratorRTWStateStorageClass=Auto  FilterContinuousStateAttributes=''  FilterStateMustResolveToSignalObject=off  FilterRTWStateStorageClass=Auto  ParallelPVariant=InternalParameters  IdealPVariant=Disabled  IVariant=InternalParameters  DVariant=Disabled  IntegratorVariant=Discrete  SatVariant=Disabled  AWVariant=Passthrough  PCopyVariant=Disabled  TRVariant=Disabled  FdbkBlocksVariant=Forward  IdealPFdbkVariant=Disabled  SatFdbkVariant=Disabled  DerivativeFilterVariant=Disabled  NVariant=Disabled  NCopyVariant=Disabled_SignalSpec  FilterICVariant=Disabled  IntegratorICVariant=InternalICs  ExternalResetVariant=Disabled  TRSumVariant=Passthrough  SumFdbkVariant=Disabled  SumVariant=Sum_PI  TsampFilterVariant=InternalTs  TsampNgainVariant=Passthrough  TsampIntegralVariant=Passthrough  ExternalSaturationOutDataTypeStr=Inherit: Same as second input
  Gain : Gain  Gain=-1
  Id_ref : Outport
  wires:
  Add/1 -> Gain/1
  Discrete PID Controller/1 -> Id_ref/1
  Gain/1 -> Discrete PID Controller/1
  Vdc_ref/1 -> Add/1
  Vdc_mea/1 -> Add/2

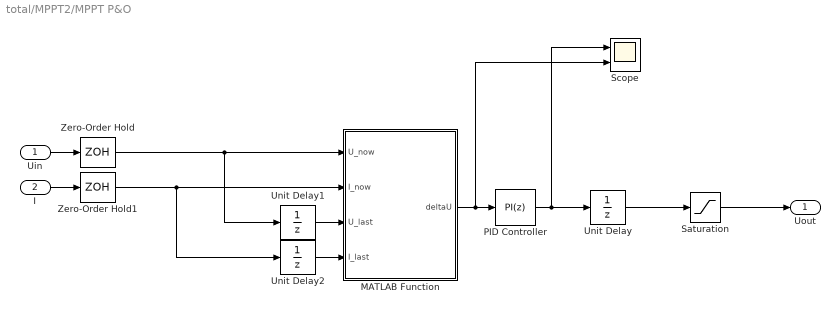
== system total/MPPT2/MPPT P&O ==
  Uin : Inport
  I : Inport  Port=2
  MATLAB Function : MATLAB Function  TreatAsAtomicUnit=on
  PID Controller : pid_lib/PID Controller  Controller=PI  Form=Parallel  TimeDomain=Discrete-time  UseExternalTs=off  SampleTime=1e-3  IntegratorMethod=Forward Euler  FilterMethod=Forward Euler  ControllerParametersSource=internal  P=1  I=100  D=0  UseFilter=on  N=100  TunerSelectOption=Transfer Function Based (PID Tuner App)  InitialConditionSource=internal  InitialConditionForIntegrator=250  InitialConditionForFilter=0  DifferentiatorICPrevScaledInput=0  ExternalReset=none  TrackingMode=off  Kt=1  LimitOutput=off  SatLimitsSource=internal  UpperSaturationLimit=inf  LowerSaturationLimit=-inf  LinearizeAsGain=on  AntiWindupMode=none  Kb=1  POutMin=[]  POutMax=[]  IOutMin=[]  IOutMax=[]  DOutMin=[]  DOutMax=[]  NOutMin=[]  NOutMax=[]  SumOutMin=[]  SumOutMax=[]  SaturationOutMin=[]  SaturationOutMax=[]  PParamMin=[]  PParamMax=[]  IParamMin=[]  IParamMax=[]  DParamMin=[]  DParamMax=[]  NParamMin=[]  NParamMax=[]  KbParamMin=[]  KbParamMax=[]  KtParamMin=[]  KtParamMax=[]  KbOutMin=[]  KbOutMax=[]  KtOutMin=[]  KtOutMax=[]  IntegratorOutMin=[]  IntegratorOutMax=[]  FilterOutMin=[]  FilterOutMax=[]  SumI1OutMin=[]  SumI1OutMax=[]  SumI2OutMin=[]  SumI2OutMax=[]  SumI3OutMin=[]  SumI3OutMax=[]  SumI4OutMin=[]  SumI4OutMax=[]  SumDOutMin=[]  SumDOutMax=[]  DifferentiatorOutMin=[]  DifferentiatorOutMax=[]  FilterDiffOutCoefMin=[]  FilterDiffOutCoefMax=[]  ReciprocalOutMin=[]  ReciprocalOutMax=[]  SumDenOutMin=[]  SumDenOutMax=[]  SumNumOutMin=[]  SumNumOutMax=[]  DivideOutMin=[]  DivideOutMax=[]  UdiffTsProdOutMin=[]  UdiffTsProdOutMax=[]  NTsProdOutMin=[]  NTsProdOutMax=[]  UintegralTsProdOutMin=[]  UintegralTsProdOutMax=[]  UngainTsProdOutMin=[]  UngainTsProdOutMax=[]  IntegratorContinuousStateAttributes=''  IntegratorStateMustResolveToSignalObject=off  IntegratorRTWStateStorageClass=Auto  FilterContinuousStateAttributes=''  FilterStateMustResolveToSignalObject=off  FilterRTWStateStorageClass=Auto  ParallelPVariant=InternalParameters  IdealPVariant=Disabled  IVariant=InternalParameters  DVariant=Disabled  IntegratorVariant=Discrete  SatVariant=Disabled  AWVariant=Passthrough  PCopyVariant=Disabled  TRVariant=Disabled  FdbkBlocksVariant=Forward  IdealPFdbkVariant=Disabled  SatFdbkVariant=Disabled  DerivativeFilterVariant=Disabled  NVariant=Disabled  NCopyVariant=Disabled_SignalSpec  FilterICVariant=Disabled  IntegratorICVariant=InternalICs  ExternalResetVariant=Disabled  TRSumVariant=Passthrough  SumFdbkVariant=Disabled  SumVariant=Sum_PI  TsampFilterVariant=InternalTs  TsampNgainVariant=Passthrough  TsampIntegralVariant=Passthrough  ExternalSaturationOutDataTypeStr=Inherit: Same as second input
  Saturation : Saturate  UpperLimit=360  LowerLimit=0
  Scope : Scope  NumInputPorts=2
  Unit Delay : UnitDelay  InitialCondition=250  SampleTime=1e-3  HasFrameUpgradeWarning=on
  Unit Delay1 : UnitDelay  InitialCondition=250  SampleTime=1e-3  HasFrameUpgradeWarning=on
  Unit Delay2 : UnitDelay  SampleTime=1e-3  HasFrameUpgradeWarning=on
  Zero-Order Hold : ZeroOrderHold  SampleTime=1e-3
  Zero-Order Hold1 : ZeroOrderHold  SampleTime=1e-3
  Uout : Outport
  wires:
  Unit Delay1/1 -> MATLAB Function/3(U_last)
  MATLAB Function/1(deltaU) -> PID Controller/1, Scope/2
  Unit Delay2/1 -> MATLAB Function/4(I_last)
  Unit Delay/1 -> Saturation/1
  Saturation/1 -> Uout/1
  I/1 -> Zero-Order Hold1/1
  Zero-Order Hold1/1 -> Unit Delay2/1, MATLAB Function/2(I_now)
  Uin/1 -> Zero-Order Hold/1
  Zero-Order Hold/1 -> Unit Delay1/1, MATLAB Function/1(U_now)
  PID Controller/1 -> Unit Delay/1, Scope/1

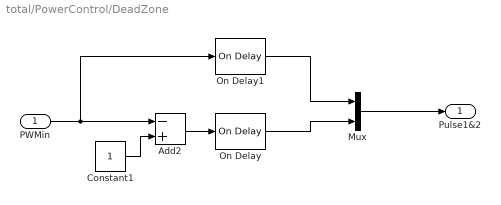
== system total/PowerControl/DeadZone ==
  PWMin : Inport
  Add2 : Sum  Inputs=-+
  Constant1 : Constant
  Mux : Mux  Inputs=2
  On Delay : spsOnDelayLib/On Delay  DelayType=On delay  delay=2e-6  ic=0  Ts=0
      settings: SourceProductBaseCode=PS
  On Delay1 : spsOnDelayLib/On Delay  DelayType=On delay  delay=2e-6  ic=0  Ts=0
      settings: SourceProductBaseCode=PS
  Pulse1&2 : Outport
  wires:
  Constant1/1 -> Add2/2
  PWMin/1 -> Add2/1, On Delay1/1
  Add2/1 -> On Delay/1
  Mux/1 -> Pulse1&2/1
  On Delay1/1 -> Mux/1
  On Delay/1 -> Mux/2

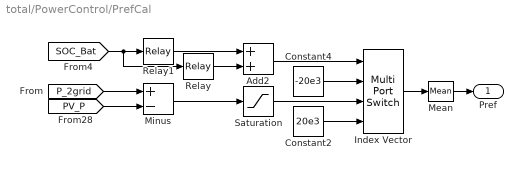
== system total/PowerControl/PrefCal ==
  Add2 : Sum
  Constant2 : Constant  Value=20e3
  Constant4 : Constant  Value=-20e3
  Index Vector : MultiPortSwitch  DataPortOrder=Zero-based contiguous  zeroidx=on
  Mean : spsMeanLib/Mean  Freq=1e4  Vinit=0  Ts=2e-6
  Minus : Sum  Inputs=+-
  Relay : Relay  OnSwitchValue=30  OffSwitchValue=10
  Relay1 : Relay  OnSwitchValue=90  OffSwitchValue=70
  Saturation : Saturate  UpperLimit=20e3  LowerLimit=-20e3
  Pref : Outport
  wires:
  Add2/1 -> Index Vector/1
  Saturation/1 -> Index Vector/3
  Minus/1 -> Saturation/1
  Index Vector/1 -> Mean/1
  [SOC_Bat] -> Relay/1, Relay1/1
  Relay/1 -> Add2/2
  Relay1/1 -> Add2/1
  Constant2/1 -> Index Vector/4
  Constant4/1 -> Index Vector/2
  [P_2grid] -> Minus/1
  [PV_P] -> Minus/2
  Mean/1 -> Pref/1

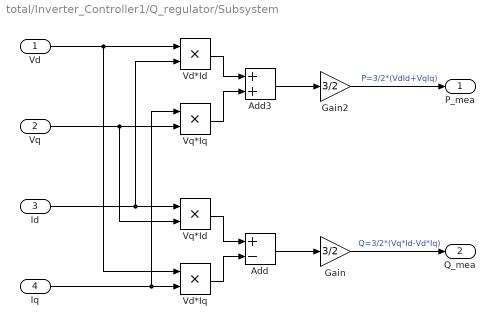
== system total/Inverter_Controller1/Q_regulator/Subsystem ==
  Vd : Inport
  Vq : Inport  Port=2
  Id : Inport  Port=3
  Iq : Inport  Port=4
  Add : Sum  Inputs=+-
  Add3 : Sum
  Gain : Gain  Gain=3/2
  Gain2 : Gain  Gain=3/2
  Vd*Id : Product
  Vd*Iq : Product
  Vq*Id : Product
  Vq*Iq : Product
  P_mea : Outport
  Q_mea : Outport  Port=2
  wires:
  Vq*Iq/1 -> Add3/2
  Add/1 -> Gain/1
  Vd*Id/1 -> Add3/1
  Id/1 -> Vd*Id/2, Vq*Id/1
  Add3/1 -> Gain2/1
  Iq/1 -> Vq*Iq/1, Vd*Iq/2
  Vd*Iq/1 -> Add/2
  Vq/1 -> Vq*Id/2, Vq*Iq/2
  Vd/1 -> Vd*Iq/1, Vd*Id/1
  Vq*Id/1 -> Add/1
  Gain2/1 -> P_mea/1  "P=3/2*(VdId+VqIq)"
  Gain/1 -> Q_mea/1  "Q=3/2*(Vq*Id-Vd*Iq)"

== matlab function total/MPPT2/MPPT P&O/MATLAB Function ==
  data: U_now input; deltaU output; I_now input; U_last input; I_last input
function deltaU  = MPPT_PandO(U_now, I_now, U_last, I_last)
    step = 5;
    %计算dP、dU
    dU = U_now - U_last;
    dP = U_now*I_now - U_last*I_last;
    
    if(dP == 0)
        deltaU = 0;
    else
        if(dP > 0)
            if(dU > 0)
                deltaU = 0 + step;
            else
                deltaU = 0 - step;
            end
        else
            if(dU > 0)
                deltaU = 0 - step;
            else
                deltaU = 0 + step;
            end
        end
    end
%     
%     if(dP == 0)
%         U_ref = U_now;
%     else
%         if(dP > 0)
%             if(dU > 0)
%                 U_ref = U_now + step;
%             else
%                 U_ref = U_now - step;
%             end
%         else
%             if(dU > 0)
%                 U_ref = U_now - step;
%             else
%                 U_ref = U_now + step;
%             end
%         end
%     end
